simulink model "rocket"  (R2025b)
settings: Solver=VariableStepAuto  StartTime=0.0  StopTime=100  MaxStep=1e-3  RelTol=1e-3
libraries: simulink x1
settings Model: SimulationMode=rapid-accelerator  Creator=123  LastModifiedBy=123

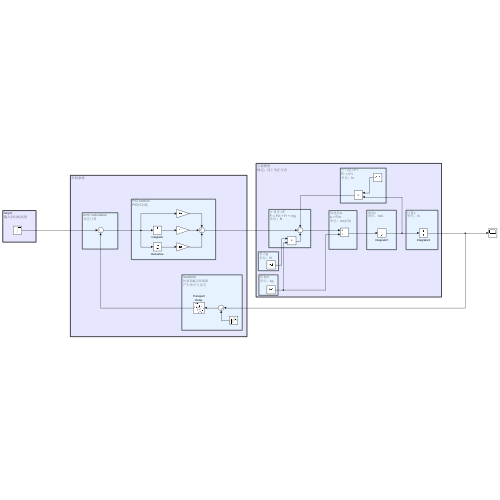
[thumbnail: Simulink's stored preview of the top-level diagram]
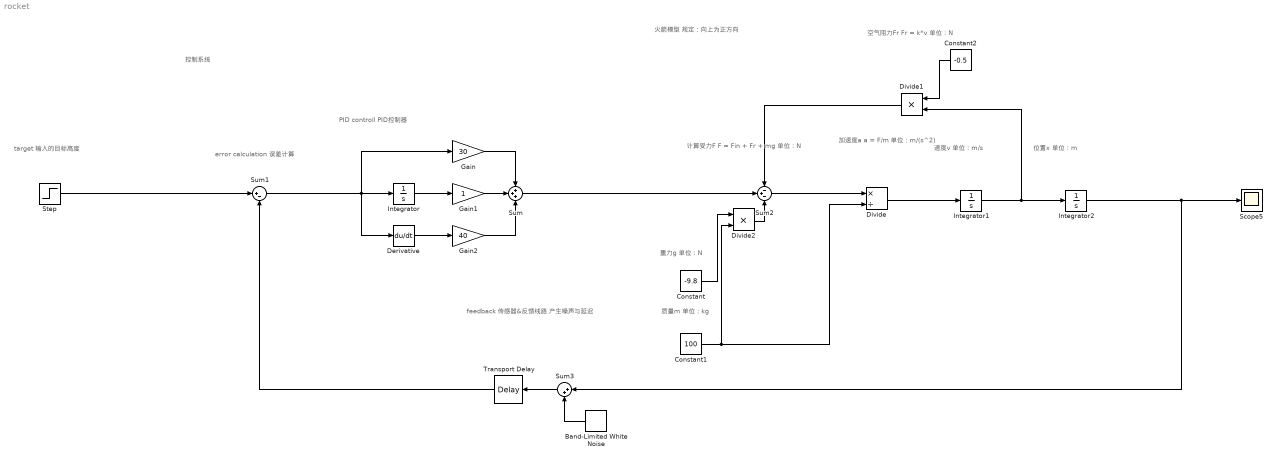
== system rocket ==
  note: 重力g
      | 单位：N
  note: 速度v
      | 单位：m/s
  note: 空气阻力Fr
      | Fr = k*v
      | 单位：N
  note: 计算受力F
      | F = Fin + Fr + mg
      | 单位：N
  note: 火箭模型
      | 规定：向上为正方向
  note: 质量m
      | 单位：kg
  note: 控制系统
  note: feedback
      | 传感器&反馈线路
      | 产生噪声与延迟
  note: error calculation
      | 误差计算
  note: 位置x
      | 单位：m
  note: target
      | 输入的目标高度
  note: 加速度a
      | a = F/m
      | 单位：m/(s^2)
  note: PID controll
      | PID控制器
  Band-Limited White Noise : simulink/Sources/Band-Limited White Noise  Cov=[0.001]  Ts=1e-3  seed=[23341]
  Constant : Constant  Value=-9.8
  Constant1 : Constant  Value=100
  Constant2 : Constant  Value=-0.5
  Derivative : Derivative
  Divide : Product  Inputs=*/
  Divide1 : Product  Inputs=**
  Divide2 : Product  Inputs=**
  Gain : Gain  Gain=30
  Gain1 : Gain
  Gain2 : Gain  Gain=40
  Integrator : Integrator
  Integrator1 : Integrator
  Integrator2 : Integrator
  Scope5 : Scope
      settings: ActiveDisplayYMinimum=-31.46773585638477  ActiveDisplayYMaximum=66.442306319999318  DataLoggingVariableName=ScopeData5
  Step : Step  After=10  SampleTime=0
  Sum : Sum  Inputs=+++
  Sum1 : Sum  Inputs=|+-
  Sum2 : Sum  Inputs=-+-
  Sum3 : Sum  Inputs=|++
  Transport Delay : TransportDelay  DelayTime=0.01  BufferSize=1024*4
  wires:
  Constant/1 -> Divide2/1
  Sum2/1 -> Divide/1
  Sum/1 -> Sum2/2
  Divide/1 -> Integrator1/1
  Gain/1 -> Sum/1
  Constant2/1 -> Divide1/1
  Integrator1/1 -> Divide1/2, Integrator2/1
  Sum1/1 -> Gain/1, Integrator/1, Derivative/1
  Gain2/1 -> Sum/3
  Step/1 -> Sum1/1
  Derivative/1 -> Gain2/1
  Gain1/1 -> Sum/2
  Integrator/1 -> Gain1/1
  Transport Delay/1 -> Sum1/2
  Constant1/1 -> Divide2/2, Divide/2
  Divide1/1 -> Sum2/1
  Divide2/1 -> Sum2/3
  Sum3/1 -> Transport Delay/1
  Integrator2/1 -> Sum3/1, Scope5/1
  Band-Limited White Noise/1 -> Sum3/2
